simulink model "ex3_sim1m"  (R2022b)
settings: Solver=ode45  StartTime=0.0  StopTime=0.5  MaxStep=0.0001  RelTol=1e-3
undefined symbols (not defined in the file): bit, degs2rpm, denC, denH, mot, numC, numH, r, rpm2rads, Ts, umax
settings Model: Creator=loren  LastModifiedBy=loren
settings DataIOCC: ReturnWorkspaceOutputs=off

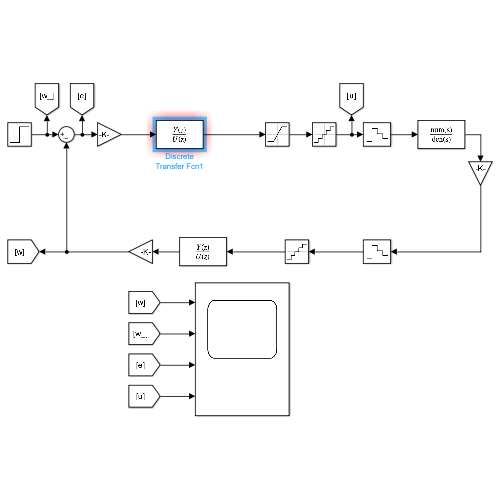
[thumbnail: Simulink's stored preview of the top-level diagram]
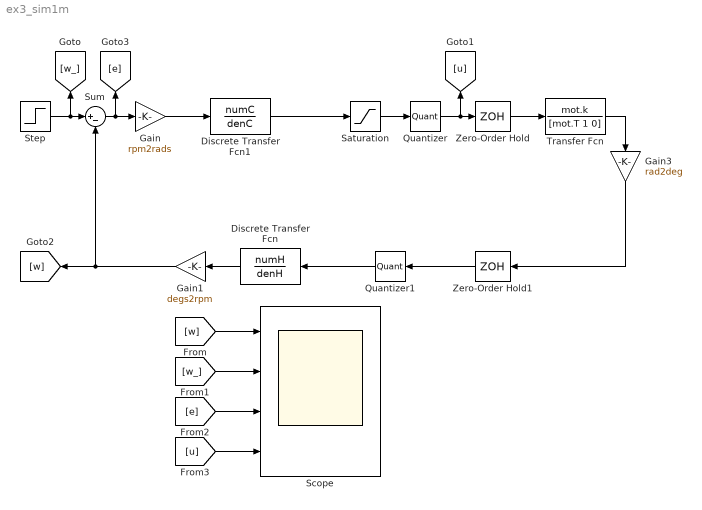
== system ex3_sim1m ==
  Discrete Transfer Fcn : DiscreteTransferFcn  Numerator=numH  Denominator=denH  SampleTime=Ts
  Discrete Transfer Fcn1 : DiscreteTransferFcn  Numerator=numC  Denominator=denC  SampleTime=Ts
  Gain : Gain  Gain=rpm2rads
  Gain1 : Gain  Gain=degs2rpm
  Gain3 : Gain  Gain=rad2deg
  Quantizer : Quantizer  QuantizationInterval=2 * umax / 2^bit
  Quantizer1 : Quantizer  QuantizationInterval=pulse2deg
  Saturation : Saturate  UpperLimit=umax  LowerLimit=-umax
  Scope : Scope  NumInputPorts=4
  Step : Step  Time=r.t  After=r.A  SampleTime=0
  Sum : Sum  Inputs=|+-
  Transfer Fcn : TransferFcn  Numerator=mot.k  Denominator=[mot.T 1 0]
  Zero-Order Hold : ZeroOrderHold  SampleTime=Ts
  Zero-Order Hold1 : ZeroOrderHold  SampleTime=Ts
  wires:
  Step/1 -> [w_], Sum/1
  Sum/1 -> [e], Gain/1
  Gain/1 -> Discrete Transfer Fcn1/1
  Discrete Transfer Fcn1/1 -> Saturation/1
  Saturation/1 -> Quantizer/1
  Quantizer/1 -> Zero-Order Hold/1, [u]
  Zero-Order Hold/1 -> Transfer Fcn/1
  Zero-Order Hold1/1 -> Quantizer1/1
  Transfer Fcn/1 -> Gain3/1
  Quantizer1/1 -> Discrete Transfer Fcn/1
  Discrete Transfer Fcn/1 -> Gain1/1
  Gain1/1 -> [w], Sum/2
  [w] -> Scope/1
  [w_] -> Scope/2
  [e] -> Scope/3
  [u] -> Scope/4
  Gain3/1 -> Zero-Order Hold1/1
